simulink model "s4dot2_25whilesubsystem"  (R2023b)
settings: Solver=VariableStepAuto  StartTime=0.0  StopTime=20  RelTol=1e-3
settings Model: Creator=lxj  LastModifiedBy=lxj

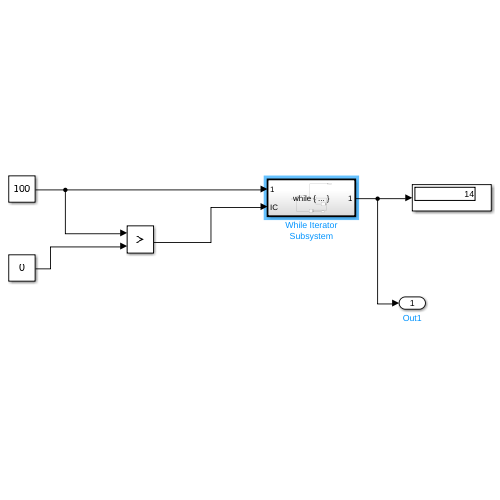
[thumbnail: Simulink's stored preview of the top-level diagram]
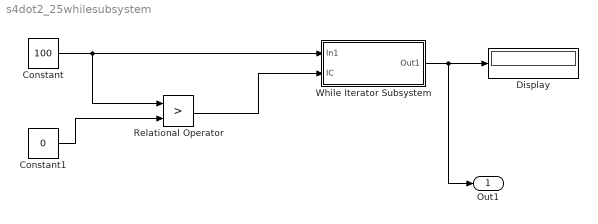
== system s4dot2_25whilesubsystem ==
  Constant : Constant  Value=100
  Constant1 : Constant  Value=0
  Display : Display
  Relational Operator : RelationalOperator  Operator=>  OutDataTypeStr=boolean  RndMeth=Simplest  InputSameDT=off
  While Iterator Subsystem : Subsystem  TreatAsAtomicUnit=on
  Out1 : Outport
  wires:
  Constant/1 -> Relational Operator/1, While Iterator Subsystem/1(In1)
  Constant1/1 -> Relational Operator/2
  Relational Operator/1 -> While Iterator Subsystem/2(IC)
  While Iterator Subsystem/1(Out1) -> Display/1, Out1/1

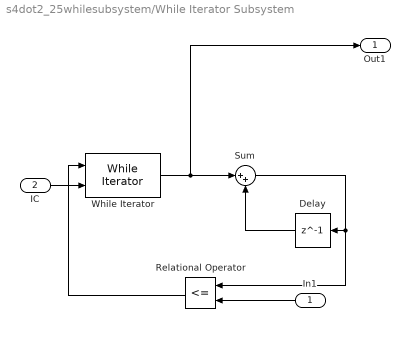
== system s4dot2_25whilesubsystem/While Iterator Subsystem ==
  In1 : Inport
  IC : Inport  Port=2
  Delay : Delay  DelayLength=1  InitialCondition=0
  Relational Operator : RelationalOperator  Operator=<=  OutDataTypeStr=boolean  RndMeth=Simplest  InputSameDT=off
  Sum : Sum  Inputs=|++
  While Iterator : WhileIterator  MaxIters=1000  ResetStates=reset  ShowIterationPort=on  OutputDataType=int16
  Out1 : Outport
  wires:
  IC/1 -> While Iterator/2
  While Iterator/1 -> Out1/1, Sum/1
  Sum/1 -> Relational Operator/1, Delay/1
  Delay/1 -> Sum/2
  In1/1 -> Relational Operator/2
  Relational Operator/1 -> While Iterator/1
